simulink model "cx06_MA"  (Simulink 7.5)
settings: Solver=FixedStepDiscrete  StartTime=0.0  StopTime=10.0  RelTol=1e-3
undefined symbols (not defined in the file or in its folder): DiscIntNeverNeededParam, ECU555, int, motohawk_build_version, motohawk_trunc_name, motohawk_vardec_path
libraries: MotoHawk_lib x811, simulink x43, simulink_need_slupdate x1
(part 9 of 10)

== system cx06_MA/Inputs/Analog Inputs/Driver Inputs/Brake ==
  2pt Calibration1_1 : Fcn  Expr=(u[1]-u[2])/(u[3]-u[2])
  2pt Calibration1_6 : Fcn  Expr=(u[1]-u[2])/(u[3]-u[2])
  Data Type Conversion2 : DataTypeConversion  OutDataTypeMode=single  OutDataType=sfix(16)  OutScaling=2^0  OutDataTypeStr=single
  Data Type Conversion5 : DataTypeConversion  OutDataTypeMode=single  OutDataType=sfix(16)  OutScaling=2^0  OutDataTypeStr=single
  Mux3 : Mux  Inputs=3
  Mux6 : Mux  Inputs=3
  Range_Detect2 : Subsystem
  Range_Detect5 : Subsystem
  Redundant_Check : Subsystem
  Saturation2 : Saturate  UpperLimit=1  LowerLimit=0
  Saturation5 : Saturate  UpperLimit=1  LowerLimit=0
  motohawk_ain2 : MotoHawk_lib/Analog I//O Blocks/motohawk_ain  res_name=[]  text_resource=AN10M  code_resource=NONE  val_resource=-1  target=ECU555-80  resource_enum_str=(None)=-1,ECUP=53,DRVP=54,XDRP=55,AN1M=56,AN2M=57,AN3M=58,AN4M=59,AN5M=60,AN6M=61,AN7M=62,AN8M=63,AN9M=64,AN10M=65,AN11M=66,AN12M=67,AN13M=68,AN14M=69,AN15M=70,AN16M=71,AN17M=72,AN18M=73,AN19M=74,O2A=90,O2B=91,XDRP_B=92  altref=5V Reference  typ=uint16  num_adc_bits=10  use_stat=on  use_vardec=on  nam='Brake'  read_level=1  write_level=1  group='I/O Pins | Inputs Config'
  motohawk_ain6 : MotoHawk_lib/Analog I//O Blocks/motohawk_ain  res_name=[]  text_resource=AN7M  code_resource=NONE  val_resource=-1  target=ECU555-80  resource_enum_str=(None)=-1,ECUP=53,DRVP=54,XDRP=55,AN1M=56,AN2M=57,AN3M=58,AN4M=59,AN5M=60,AN6M=61,AN7M=62,AN8M=63,AN9M=64,AN10M=65,AN11M=66,AN12M=67,AN13M=68,AN14M=69,AN15M=70,AN16M=71,AN17M=72,AN18M=73,AN19M=74,O2A=90,O2B=91,XDRP_B=92  altref=5V Reference  typ=uint16  num_adc_bits=10  use_stat=on  use_vardec=on  nam='BrakeBackUp'  read_level=1  write_level=1  group='I/O Pins | Inputs Config'
  motohawk_calibration1 : MotoHawk_lib/Calibration & Probing Blocks/motohawk_calibration  nam='Brake_Redun_Err'  val=1  storage=Calibration  show_more=on  name_source=Use Parameter  data_type=Inherit via back propagation  read_level=1  write_level=1  ovr_cals=on  view_as=Number  enum_struct={'Disabled', 'Enabled'}  vector_style=Wide Row  use_help_units=on  help='Brake sensors must be within this error else Redundante Fault'  units=''  use_header_enum=off  row_header_enum={}  col_header_enum={}  use_min_max=on  min_val=0  max_val=1.2  use_precision=on  precision='1.2'  gain=1  offset=0  exp=1  use_mototune_group=off  mototune_group=motohawk_vardec_path(gcb)
  motohawk_calibration11 : MotoHawk_lib/Calibration & Probing Blocks/motohawk_calibration  nam='BrakeBackup_Full'  val=597  storage=Calibration  show_more=on  name_source=Use Parameter  data_type=Inherit via back propagation  read_level=1  write_level=1  ovr_cals=on  view_as=Number  enum_struct={'Disabled', 'Enabled'}  vector_style=Wide Row  use_help_units=off  help=''  units=''  use_header_enum=off  row_header_enum={}  col_header_enum={}  use_min_max=off  min_val=-inf  max_val=inf  use_precision=off  precision=''  gain=1  offset=0  exp=1  use_mototune_group=off  mototune_group=motohawk_vardec_path(gcb)
  motohawk_calibration12 : MotoHawk_lib/Calibration & Probing Blocks/motohawk_calibration  nam='BrakeBackup_Zero'  val=678  storage=Calibration  show_more=on  name_source=Use Parameter  data_type=Inherit via back propagation  read_level=1  write_level=1  ovr_cals=on  view_as=Number  enum_struct={'Disabled', 'Enabled'}  vector_style=Wide Row  use_help_units=off  help=''  units=''  use_header_enum=off  row_header_enum={}  col_header_enum={}  use_min_max=off  min_val=-inf  max_val=inf  use_precision=off  precision=''  gain=1  offset=0  exp=1  use_mototune_group=off  mototune_group=motohawk_vardec_path(gcb)
  motohawk_calibration5 : MotoHawk_lib/Calibration & Probing Blocks/motohawk_calibration  nam='Brake_Zero'  val=925  storage=Calibration  show_more=on  name_source=Use Parameter  data_type=Inherit via back propagation  read_level=1  write_level=1  ovr_cals=on  view_as=Number  enum_struct={'Disabled', 'Enabled'}  vector_style=Wide Row  use_help_units=off  help=''  units=''  use_header_enum=off  row_header_enum={}  col_header_enum={}  use_min_max=off  min_val=-inf  max_val=inf  use_precision=off  precision=''  gain=1  offset=0  exp=1  use_mototune_group=off  mototune_group=motohawk_vardec_path(gcb)
  motohawk_calibration6 : MotoHawk_lib/Calibration & Probing Blocks/motohawk_calibration  nam='Brake_Full'  val=37  storage=Calibration  show_more=on  name_source=Use Parameter  data_type=Inherit via back propagation  read_level=1  write_level=1  ovr_cals=on  view_as=Number  enum_struct={'Disabled', 'Enabled'}  vector_style=Wide Row  use_help_units=off  help=''  units=''  use_header_enum=off  row_header_enum={}  col_header_enum={}  use_min_max=off  min_val=-inf  max_val=inf  use_precision=off  precision=''  gain=1  offset=0  exp=1  use_mototune_group=off  mototune_group=motohawk_vardec_path(gcb)
  motohawk_fault_def1 : MotoHawk_lib/Fault Management Blocks/motohawk_fault_def  nam='BrakeRedundant'  mode=Disabled  id=[]  x=10  y=20  input_suspected=on  indeterminate=off  increment_xy=on  downsample_count=1  ovr_cals=on  ovr_actions=on  show_actions=on  action1_name='inhibitRegen'  action1_cond=Active  action2_name=''  action2_cond=(None)  action3_name=''  action3_cond=(None)  action4_name=''  action4_cond=(None)
  motohawk_fault_def3 : MotoHawk_lib/Fault Management Blocks/motohawk_fault_def  nam='BrakeRange'  mode=Disabled  id=[]  x=10  y=20  input_suspected=on  indeterminate=off  increment_xy=on  downsample_count=1  ovr_cals=on  ovr_actions=on  show_actions=on  action1_name='inhibitRegen'  action1_cond=Active  action2_name=''  action2_cond=(None)  action3_name=''  action3_cond=(None)  action4_name=''  action4_cond=(None)
  motohawk_fault_def6 : MotoHawk_lib/Fault Management Blocks/motohawk_fault_def  nam='BrakeBackupRange'  mode=Disabled  id=[]  x=10  y=20  input_suspected=on  indeterminate=off  increment_xy=on  downsample_count=1  ovr_cals=on  ovr_actions=on  show_actions=on  action1_name='inhibitRegen'  action1_cond=Active  action2_name=''  action2_cond=(None)  action3_name=''  action3_cond=(None)  action4_name=''  action4_cond=(None)
  motohawk_probe11 : MotoHawk_lib/Calibration & Probing Blocks/motohawk_probe  nam='In_Brake'  show_more=on  name_source=Use Parameter  read_level=1  view_as=Number  enum_struct={'Disabled', 'Enabled'}  vector_style=Wide Row  use_help_units=off  help=''  units=''  use_header_enum=off  row_header_enum={}  col_header_enum={}  use_precision=off  precision=''  gain=1  offset=0  exp=1  use_mototune_group=on  mototune_group='Debug | Inputs'
  motohawk_probe17 : MotoHawk_lib/Calibration & Probing Blocks/motohawk_probe  nam='In_BrakeBackup'  show_more=on  name_source=Use Parameter  read_level=1  view_as=Number  enum_struct={'Disabled', 'Enabled'}  vector_style=Wide Row  use_help_units=off  help=''  units=''  use_header_enum=off  row_header_enum={}  col_header_enum={}  use_precision=off  precision=''  gain=1  offset=0  exp=1  use_mototune_group=on  mototune_group='Debug | Inputs'
  motohawk_probe18 : MotoHawk_lib/Calibration & Probing Blocks/motohawk_probe  nam='raw_BrakeBackup'  show_more=on  name_source=Use Parameter  read_level=1  view_as=Number  enum_struct={'Disabled', 'Enabled'}  vector_style=Wide Row  use_help_units=on  help=''  units=''  use_header_enum=off  row_header_enum={}  col_header_enum={}  use_precision=off  precision=''  gain=1  offset=0  exp=1  use_mototune_group=off  mototune_group=motohawk_vardec_path(gcb)
  motohawk_probe19 : MotoHawk_lib/Calibration & Probing Blocks/motohawk_probe  nam='cal_BrakeBackup'  show_more=on  name_source=Use Parameter  read_level=1  view_as=Number  enum_struct={'Disabled', 'Enabled'}  vector_style=Wide Row  use_help_units=off  help=''  units=''  use_header_enum=off  row_header_enum={}  col_header_enum={}  use_precision=off  precision=''  gain=1  offset=0  exp=1  use_mototune_group=off  mototune_group=motohawk_vardec_path(gcb)
  motohawk_probe5 : MotoHawk_lib/Calibration & Probing Blocks/motohawk_probe  nam='raw_Brake'  show_more=on  name_source=Use Parameter  read_level=1  view_as=Number  enum_struct={'Disabled', 'Enabled'}  vector_style=Wide Row  use_help_units=on  help=''  units=''  use_header_enum=off  row_header_enum={}  col_header_enum={}  use_precision=off  precision=''  gain=1  offset=0  exp=1  use_mototune_group=off  mototune_group=motohawk_vardec_path(gcb)
  motohawk_probe6 : MotoHawk_lib/Calibration & Probing Blocks/motohawk_probe  nam='cal_Brake'  show_more=on  name_source=Use Parameter  read_level=1  view_as=Number  enum_struct={'Disabled', 'Enabled'}  vector_style=Wide Row  use_help_units=off  help=''  units=''  use_header_enum=off  row_header_enum={}  col_header_enum={}  use_precision=off  precision=''  gain=1  offset=0  exp=1  use_mototune_group=off  mototune_group=motohawk_vardec_path(gcb)
  Brake : Outport  OutDataType=sfix(16)  OutScaling=2^0
  wires:
  motohawk_ain2/1 -> motohawk_probe5/1, Data Type Conversion2/1
  motohawk_calibration5/1 -> Mux3/2, Range_Detect2/2(Zero)
  motohawk_calibration6/1 -> Mux3/3, Range_Detect2/3(Full)
  Mux3/1 -> 2pt Calibration1_1/1
  2pt Calibration1_1/1 -> Saturation2/1
  Data Type Conversion2/1 -> Mux3/1, Range_Detect2/1(Value)
  Saturation2/1 -> motohawk_probe6/1, Redundant_Check/1(In1), Brake/1  "Brake"
  Range_Detect2/1(Fault) -> motohawk_fault_def3/1
  motohawk_ain2/2 -> motohawk_probe11/1
  motohawk_ain6/1 -> Data Type Conversion5/1, motohawk_probe18/1
  motohawk_calibration12/1 -> Mux6/2, Range_Detect5/2(Zero)
  motohawk_calibration11/1 -> Mux6/3, Range_Detect5/3(Full)
  Mux6/1 -> 2pt Calibration1_6/1
  2pt Calibration1_6/1 -> Saturation5/1
  Data Type Conversion5/1 -> Mux6/1, Range_Detect5/1(Value)
  Saturation5/1 -> motohawk_probe19/1, Redundant_Check/3(In2)  "BrakeBackup"
  Range_Detect5/1(Fault) -> motohawk_fault_def6/1
  motohawk_ain6/2 -> motohawk_probe17/1
  motohawk_calibration1/1 -> Redundant_Check/2(Allowable_Error)
  Redundant_Check/1(Fault) -> motohawk_fault_def1/1

== system cx06_MA/Inputs/Analog Inputs/Driver Inputs/Clutch ==
  2pt Calibration1_4 : Fcn  Expr=(u[1]-u[2])/(u[3]-u[2])
  2pt Calibration1_5 : Fcn  Expr=(u[1]-u[2])/(u[3]-u[2])
  Data Type Conversion3 : DataTypeConversion  OutDataTypeMode=single  OutDataType=sfix(16)  OutScaling=2^0  OutDataTypeStr=single
  Data Type Conversion4 : DataTypeConversion  OutDataTypeMode=single  OutDataType=sfix(16)  OutScaling=2^0  OutDataTypeStr=single
  Mux4 : Mux  Inputs=3
  Mux5 : Mux  Inputs=3
  Range_Detect3 : Subsystem
  Range_Detect4 : Subsystem
  Redundant_Check : Subsystem
  Saturation3 : Saturate  UpperLimit=1  LowerLimit=0
  Saturation4 : Saturate  UpperLimit=1  LowerLimit=0
  motohawk_ain3 : MotoHawk_lib/Analog I//O Blocks/motohawk_ain  res_name=[]  text_resource=AN8M  code_resource=NONE  val_resource=-1  target=ECU555-80  resource_enum_str=(None)=-1,ECUP=53,DRVP=54,XDRP=55,AN1M=56,AN2M=57,AN3M=58,AN4M=59,AN5M=60,AN6M=61,AN7M=62,AN8M=63,AN9M=64,AN10M=65,AN11M=66,AN12M=67,AN13M=68,AN14M=69,AN15M=70,AN16M=71,AN17M=72,AN18M=73,AN19M=74,O2A=90,O2B=91,XDRP_B=92  altref=5V Reference  typ=uint16  num_adc_bits=10  use_stat=on  use_vardec=on  nam='Clutch'  read_level=1  write_level=1  group='I/O Pins | Inputs Config'
  motohawk_ain5 : MotoHawk_lib/Analog I//O Blocks/motohawk_ain  res_name=[]  text_resource=(None)  code_resource=NONE  val_resource=-1  target=ECU555-80  resource_enum_str=(None)=-1,ECUP=53,DRVP=54,XDRP=55,AN1M=56,AN2M=57,AN3M=58,AN4M=59,AN5M=60,AN6M=61,AN7M=62,AN8M=63,AN9M=64,AN10M=65,AN11M=66,AN12M=67,AN13M=68,AN14M=69,AN15M=70,AN16M=71,AN17M=72,AN18M=73,AN19M=74,O2A=90,O2B=91,XDRP_B=92  altref=5V Reference  typ=uint16  num_adc_bits=10  use_stat=on  use_vardec=on  nam='ClutchBackup'  read_level=1  write_level=1  group='I/O Pins | Inputs Config'
  motohawk_calibration1 : MotoHawk_lib/Calibration & Probing Blocks/motohawk_calibration  nam='Clutch_Redun_Err'  val=1  storage=Calibration  show_more=on  name_source=Use Parameter  data_type=Inherit via back propagation  read_level=1  write_level=1  ovr_cals=on  view_as=Number  enum_struct={'Disabled', 'Enabled'}  vector_style=Wide Row  use_help_units=on  help='Brake sensors must be within this error else Redundante Fault'  units=''  use_header_enum=off  row_header_enum={}  col_header_enum={}  use_min_max=on  min_val=0  max_val=1  use_precision=on  precision='1.2'  gain=1  offset=0  exp=1  use_mototune_group=off  mototune_group=motohawk_vardec_path(gcb)
  motohawk_calibration10 : MotoHawk_lib/Calibration & Probing Blocks/motohawk_calibration  nam='ClutchBackup_Full'  val=.75  storage=Calibration  show_more=on  name_source=Use Parameter  data_type=Inherit via back propagation  read_level=1  write_level=1  ovr_cals=on  view_as=Number  enum_struct={'Disabled', 'Enabled'}  vector_style=Wide Row  use_help_units=off  help=''  units=''  use_header_enum=off  row_header_enum={}  col_header_enum={}  use_min_max=off  min_val=-inf  max_val=inf  use_precision=off  precision=''  gain=1  offset=0  exp=1  use_mototune_group=off  mototune_group=motohawk_vardec_path(gcb)
  motohawk_calibration7 : MotoHawk_lib/Calibration & Probing Blocks/motohawk_calibration  nam='Clutch_Zero'  val=110  storage=Calibration  show_more=on  name_source=Use Parameter  data_type=Inherit via back propagation  read_level=1  write_level=1  ovr_cals=on  view_as=Number  enum_struct={'Disabled', 'Enabled'}  vector_style=Wide Row  use_help_units=off  help=''  units=''  use_header_enum=off  row_header_enum={}  col_header_enum={}  use_min_max=off  min_val=-inf  max_val=inf  use_precision=off  precision=''  gain=1  offset=0  exp=1  use_mototune_group=off  mototune_group=motohawk_vardec_path(gcb)
  motohawk_calibration8 : MotoHawk_lib/Calibration & Probing Blocks/motohawk_calibration  nam='Clutch_Full'  val=1015  storage=Calibration  show_more=on  name_source=Use Parameter  data_type=Inherit via back propagation  read_level=1  write_level=1  ovr_cals=on  view_as=Number  enum_struct={'Disabled', 'Enabled'}  vector_style=Wide Row  use_help_units=off  help=''  units=''  use_header_enum=off  row_header_enum={}  col_header_enum={}  use_min_max=off  min_val=-inf  max_val=inf  use_precision=off  precision=''  gain=1  offset=0  exp=1  use_mototune_group=off  mototune_group=motohawk_vardec_path(gcb)
  motohawk_calibration9 : MotoHawk_lib/Calibration & Probing Blocks/motohawk_calibration  nam='ClutchBackup_Zero'  val=.5  storage=Calibration  show_more=on  name_source=Use Parameter  data_type=Inherit via back propagation  read_level=1  write_level=1  ovr_cals=on  view_as=Number  enum_struct={'Disabled', 'Enabled'}  vector_style=Wide Row  use_help_units=off  help=''  units=''  use_header_enum=off  row_header_enum={}  col_header_enum={}  use_min_max=off  min_val=-inf  max_val=inf  use_precision=off  precision=''  gain=1  offset=0  exp=1  use_mototune_group=off  mototune_group=motohawk_vardec_path(gcb)
  motohawk_fault_def1 : MotoHawk_lib/Fault Management Blocks/motohawk_fault_def  nam='ClutchRedundant'  mode=Sticky  id=[]  x=10  y=20  input_suspected=on  indeterminate=off  increment_xy=on  downsample_count=1  ovr_cals=on  ovr_actions=on  show_actions=on  action1_name='inhibitEngineSS'  action1_cond=Active  action2_name='inhibitAssistTakeoff'  action2_cond=(None)  action3_name='Clutch'  action3_cond=(None)  action4_name=''  action4_cond=(None)
  motohawk_fault_def4 : MotoHawk_lib/Fault Management Blocks/motohawk_fault_def  nam='ClutchRange'  mode=Disabled  id=[]  x=10  y=20  input_suspected=on  indeterminate=off  increment_xy=on  downsample_count=1  ovr_cals=on  ovr_actions=on  show_actions=on  action1_name='inhibitEngineSS'  action1_cond=Active  action2_name='inhibitAssistTakeoff'  action2_cond=Active  action3_name='Clutch'  action3_cond=Active  action4_name=''  action4_cond=(None)
  motohawk_fault_def5 : MotoHawk_lib/Fault Management Blocks/motohawk_fault_def  nam='ClutchBackupRange'  mode=Disabled  id=[]  x=10  y=20  input_suspected=on  indeterminate=off  increment_xy=on  downsample_count=1  ovr_cals=on  ovr_actions=on  show_actions=on  action1_name='inhibitEngineSS'  action1_cond=Active  action2_name='inhibitAssistTakeoff'  action2_cond=Active  action3_name='Clutch'  action3_cond=Active  action4_name=''  action4_cond=(None)
  motohawk_probe12 : MotoHawk_lib/Calibration & Probing Blocks/motohawk_probe  nam='In_Clutch'  show_more=on  name_source=Use Parameter  read_level=1  view_as=Number  enum_struct={'Disabled', 'Enabled'}  vector_style=Wide Row  use_help_units=off  help=''  units=''  use_header_enum=off  row_header_enum={}  col_header_enum={}  use_precision=off  precision=''  gain=1  offset=0  exp=1  use_mototune_group=on  mototune_group='Debug | Inputs'
  motohawk_probe13 : MotoHawk_lib/Calibration & Probing Blocks/motohawk_probe  nam='In_ClutchBackup'  show_more=on  name_source=Use Parameter  read_level=1  view_as=Number  enum_struct={'Disabled', 'Enabled'}  vector_style=Wide Row  use_help_units=off  help=''  units=''  use_header_enum=off  row_header_enum={}  col_header_enum={}  use_precision=off  precision=''  gain=1  offset=0  exp=1  use_mototune_group=on  mototune_group='Debug | Inputs'
  motohawk_probe14 : MotoHawk_lib/Calibration & Probing Blocks/motohawk_probe  nam='raw_ClutchBackup'  show_more=on  name_source=Use Parameter  read_level=1  view_as=Number  enum_struct={'Disabled', 'Enabled'}  vector_style=Wide Row  use_help_units=on  help=''  units=''  use_header_enum=off  row_header_enum={}  col_header_enum={}  use_precision=off  precision=''  gain=1  offset=0  exp=1  use_mototune_group=off  mototune_group=motohawk_vardec_path(gcb)
  motohawk_probe15 : MotoHawk_lib/Calibration & Probing Blocks/motohawk_probe  nam='cal_ClutchBackup'  show_more=on  name_source=Use Parameter  read_level=1  view_as=Number  enum_struct={'Disabled', 'Enabled'}  vector_style=Wide Row  use_help_units=off  help=''  units=''  use_header_enum=off  row_header_enum={}  col_header_enum={}  use_precision=off  precision=''  gain=1  offset=0  exp=1  use_mototune_group=off  mototune_group=motohawk_vardec_path(gcb)
  motohawk_probe7 : MotoHawk_lib/Calibration & Probing Blocks/motohawk_probe  nam='raw_Clutch'  show_more=on  name_source=Use Parameter  read_level=1  view_as=Number  enum_struct={'Disabled', 'Enabled'}  vector_style=Wide Row  use_help_units=on  help=''  units=''  use_header_enum=off  row_header_enum={}  col_header_enum={}  use_precision=off  precision=''  gain=1  offset=0  exp=1  use_mototune_group=off  mototune_group=motohawk_vardec_path(gcb)
  motohawk_probe8 : MotoHawk_lib/Calibration & Probing Blocks/motohawk_probe  nam='cal_Clutch'  show_more=on  name_source=Use Parameter  read_level=1  view_as=Number  enum_struct={'Disabled', 'Enabled'}  vector_style=Wide Row  use_help_units=off  help=''  units=''  use_header_enum=off  row_header_enum={}  col_header_enum={}  use_precision=off  precision=''  gain=1  offset=0  exp=1  use_mototune_group=off  mototune_group=motohawk_vardec_path(gcb)
  Clutch : Outport  OutDataType=sfix(16)  OutScaling=2^0
  wires:
  motohawk_ain3/1 -> Data Type Conversion3/1, motohawk_probe7/1
  motohawk_calibration7/1 -> Mux4/2, Range_Detect3/2(Zero)
  motohawk_calibration8/1 -> Mux4/3, Range_Detect3/3(Full)
  Mux4/1 -> 2pt Calibration1_4/1
  2pt Calibration1_4/1 -> Saturation3/1
  Data Type Conversion3/1 -> Mux4/1, Range_Detect3/1(Value)
  Saturation3/1 -> motohawk_probe8/1, Redundant_Check/1(In1), Clutch/1  "Clutch"
  Range_Detect3/1(Fault) -> motohawk_fault_def4/1
  motohawk_ain3/2 -> motohawk_probe12/1
  motohawk_ain5/1 -> Data Type Conversion4/1, motohawk_probe14/1
  motohawk_calibration9/1 -> Mux5/2, Range_Detect4/2(Zero)
  motohawk_calibration10/1 -> Mux5/3, Range_Detect4/3(Full)
  Mux5/1 -> 2pt Calibration1_5/1
  2pt Calibration1_5/1 -> Saturation4/1
  Data Type Conversion4/1 -> Mux5/1, Range_Detect4/1(Value)
  Saturation4/1 -> motohawk_probe15/1, Redundant_Check/3(In2)  "ClutchBackup"
  Range_Detect4/1(Fault) -> motohawk_fault_def5/1
  motohawk_ain5/2 -> motohawk_probe13/1
  motohawk_calibration1/1 -> Redundant_Check/2(Allowable_Error)
  Redundant_Check/1(Fault) -> motohawk_fault_def1/1

== system cx06_MA/Inputs/Analog Inputs/Fuel Level/Range_Detect ==
  Value : Inport  OutDataType=sfix(16)  OutScaling=2^0
  Zero : Inport  Port=2  OutDataType=sfix(16)  OutScaling=2^0
  Full : Inport  Port=3  OutDataType=sfix(16)  OutScaling=2^0
  Gain : Gain  Gain=0.1  ParameterDataType=sfix(16)  ParameterScaling=2^0  OutDataType=sfix(16)  OutScaling=2^0
  Logical Operator : Logic  Operator=OR  AllPortsSameDT=off  OutDataTypeMode=boolean  OutDataTypeStr=boolean
  MinMax : MinMax  Inputs=2  OutDataType=sfix(16)  OutScaling=2^0
  MinMax1 : MinMax  Function=max  Inputs=2  OutDataType=sfix(16)  OutScaling=2^0
  Relational Operator : RelationalOperator  Operator=>  LogicOutDataTypeMode=boolean  OutDataTypeStr=boolean
  Relational Operator1 : RelationalOperator  Operator=>  LogicOutDataTypeMode=boolean  OutDataTypeStr=boolean
  Sum : Sum  Inputs=|+-  OutDataType=sfix(16)  OutScaling=2^0
  Sum1 : Sum  Inputs=-+  OutDataType=sfix(16)  OutScaling=2^0
  Sum2 : Sum  Inputs=++|  OutDataType=sfix(16)  OutScaling=2^0
  Fault : Outport  OutDataType=sfix(16)  OutScaling=2^0
  wires:
  Zero/1 -> MinMax/1, MinMax1/2
  Full/1 -> MinMax/2, MinMax1/1
  MinMax/1 -> Sum1/1, Sum/1
  MinMax1/1 -> Sum1/2, Sum2/2
  Sum1/1 -> Gain/1
  Gain/1 -> Sum/2, Sum2/1
  Sum2/1 -> Relational Operator1/2
  Sum/1 -> Relational Operator/1
  Value/1 -> Relational Operator/2, Relational Operator1/1
  Relational Operator/1 -> Logical Operator/1
  Relational Operator1/1 -> Logical Operator/2
  Logical Operator/1 -> Fault/1

== system cx06_MA/Outputs/Analog Outputs/Backup_Relay_Control/Subsystem ==
  timer_en : Inport  OutDataType=sfix(16)  OutScaling=2^0
  Idle_to_Crank Cal : Inport  Port=2  OutDataType=sfix(16)  OutScaling=2^0
  Crank_to_Idle Cal : Inport  Port=3  OutDataType=sfix(16)  OutScaling=2^0
  Constant : Constant  Value=0  OutDataType=sfix(16)  OutScaling=2^0
  Constant1 : Constant  OutDataType=sfix(16)  OutScaling=2^0
  Relational Operator : RelationalOperator  LogicOutDataTypeMode=boolean  OutDataTypeStr=boolean
  Relational Operator1 : RelationalOperator  Operator=<=  LogicOutDataTypeMode=boolean  OutDataTypeStr=boolean
  Saturation : Saturate  UpperLimit=300  LowerLimit=0
  Sum : Sum  Inputs=|++  OutDataType=sfix(16)  OutScaling=2^0
  Switch1 : Switch  Criteria=u2 > Threshold  OutDataTypeStr=Inherit: Inherit via back propagation
  Unit Delay : UnitDelay  SampleTime=-1
  Timer : Outport  OutDataType=sfix(16)  OutScaling=2^0
  Idle_to_Crank Delay : Outport  Port=2  OutDataType=sfix(16)  OutScaling=2^0
  Crank_to_Idle Delay : Outport  Port=3  OutDataType=sfix(16)  OutScaling=2^0
  wires:
  Switch1/1 -> Saturation/1
  Saturation/1 -> Timer/1, Relational Operator/1, Unit Delay/1, Relational Operator1/2
  Constant/1 -> Switch1/3
  Constant1/1 -> Sum/2
  Sum/1 -> Switch1/1
  timer_en/1 -> Switch1/2
  Crank_to_Idle Cal/1 -> Relational Operator/2
  Relational Operator/1 -> Crank_to_Idle Delay/1
  Idle_to_Crank Cal/1 -> Relational Operator1/1
  Relational Operator1/1 -> Idle_to_Crank Delay/1
  Unit Delay/1 -> Sum/1

== system cx06_MA/Outputs/GMLAN Outputs/Fuel/SOC_Gage_Conditioning/Fuel_Signal_Conditioning ==
  note: Regular Filter to keep fuel gage from "bouncing" around;
      | also, on start up, it passes though the unfiltered value
  Fuel_Level : Inport  OutDataType=sfix(16)  OutScaling=2^0
  Constant : Constant  OutDataType=sfix(16)  OutScaling=2^0
  Gain : Gain  Gain=100  ParameterDataType=sfix(16)  ParameterScaling=2^0  OutDataType=sfix(16)  OutScaling=2^0
  Product : Product  OutDataType=sfix(16)  OutScaling=2^0  RndMeth=Zero
  Product1 : Product  OutDataType=sfix(16)  OutScaling=2^0  RndMeth=Zero
  Sum : Sum  Inputs=|++  OutDataType=sfix(16)  OutScaling=2^0
  Sum1 : Sum  Inputs=|-+  OutDataType=sfix(16)  OutScaling=2^0
  Switch : Switch  Criteria=u2 > Threshold  Threshold=-1
  Unit Delay1 : UnitDelay  X0=-1  SampleTime=-1
  motohawk_calibration : MotoHawk_lib/Calibration & Probing Blocks/motohawk_calibration  nam='Fuel_Filter_K'  val=.0001  storage=Calibration  show_more=on  name_source=Use Parameter  data_type=Inherit from 'Default Value'  read_level=1  write_level=1  ovr_cals=on  view_as=Number  enum_struct={'Disabled', 'Enabled'}  vector_style=Wide Row  use_help_units=off  help=''  units=''  use_header_enum=off  row_header_enum={}  col_header_enum={}  use_min_max=on  min_val=0  max_val=1  use_precision=on  precision='1.4'  gain=1  offset=0  exp=1  use_mototune_group=off  mototune_group=motohawk_vardec_path(gcb)
  Out1 : Outport  OutDataType=sfix(16)  OutScaling=2^0
  wires:
  motohawk_calibration/1 -> Product/2, Sum1/1
  Product/1 -> Sum/1
  Constant/1 -> Sum1/2
  Sum1/1 -> Product1/1
  Product1/1 -> Sum/2
  Unit Delay1/1 -> Product1/2, Switch/2
  Sum/1 -> Switch/1
  Gain/1 -> Product/1, Switch/3
  Switch/1 -> Out1/1, Unit Delay1/1
  Fuel_Level/1 -> Gain/1

== system cx06_MA/Strategy/Hybrid Control Code/Activation of Traction Control/RRef_Wheel Diff ==
  Inputs : Inport  OutDataType=sfix(16)  OutScaling=2^0
  Action Port : ActionPort  ActionType=case
  Abs{1..4} (4 alike) : Abs
  Bus Selector : BusSelector  OutputSignals=GMLAN.FL_Whl_Spd,GMLAN.FR_Whl_Spd,GMLAN.RL_Whl_Spd,GMLAN.RR_Whl_Spd
  Logical Operator : Logic  Operator=OR  AllPortsSameDT=off  OutDataTypeMode=Specify via dialog  OutDataTypeStr=uint(8)
  MinMax : MinMax  Inputs=2  OutDataType=sfix(16)  OutScaling=2^0
  MinMax1 : MinMax  Function=max  Inputs=2  OutDataType=sfix(16)  OutScaling=2^0
  MinMax2 : MinMax  Function=max  Inputs=2  OutDataType=sfix(16)  OutScaling=2^0
  MinMax3 : MinMax  Inputs=2  OutDataType=sfix(16)  OutScaling=2^0
  Relational Operator1 : RelationalOperator  Operator=>  LogicOutDataTypeMode=Specify via dialog  OutDataTypeStr=uint(8)
  Relational Operator2 : RelationalOperator  Operator=>  LogicOutDataTypeMode=Specify via dialog  OutDataTypeStr=uint(8)
  Relational Operator3 : RelationalOperator  Operator=>  LogicOutDataTypeMode=Specify via dialog  OutDataTypeStr=uint(8)
  Sum1 : Sum  Inputs=+-  OutDataType=sfix(16)  OutScaling=2^0
  Sum2 : Sum  Inputs=-+  OutDataType=sfix(16)  OutScaling=2^0
  Sum3 : Sum  Inputs=+-  OutDataType=sfix(16)  OutScaling=2^0
  motohawk_calibration : MotoHawk_lib/Calibration & Probing Blocks/motohawk_calibration  nam='TC_Slip_Thres'  val=10  storage=Calibration  show_more=on  name_source=Use Parameter  data_type=Inherit from 'Default Value'  read_level=1  write_level=1  ovr_cals=on  view_as=Number  enum_struct={'Disabled', 'Enabled'}  vector_style=Wide Row  use_help_units=on  help='max allowable wheel spd difference before TC become active'  units='rpm'  use_header_enum=off  row_header_enum={}  col_header_enum={}  use_min_max=on  min_val=0  max_val=inf  use_precision=off  precision=''  gain=1  offset=0  exp=1  use_mototune_group=off  mototune_group=motohawk_vardec_path(gcb)
  Front_Slip? : Outport  OutDataType=sfix(16)  OutScaling=2^0
  Rear_Slip? : Outport  Port=2  OutDataType=sfix(16)  OutScaling=2^0
  wires:
  Inputs/1 -> Bus Selector/1
  Bus Selector/3 -> Abs1/1  "<RL_Whl_Spd>"
  Bus Selector/4 -> Abs2/1  "<RR_Whl_Spd>"
  Abs1/1 -> MinMax/1
  Abs2/1 -> MinMax/2, MinMax2/1, MinMax2/2
  Bus Selector/2 -> Abs3/1  "<FR_Whl_Spd>"
  MinMax/1 -> Sum1/2, Sum2/1
  Bus Selector/1 -> Abs4/1  "<FL_Whl_Spd>"
  Sum1/1 -> Relational Operator2/1
  motohawk_calibration/1 -> Relational Operator2/2, Relational Operator1/2, Relational Operator3/2
  Relational Operator2/1 -> Front_Slip?/1
  Abs4/1 -> MinMax1/1, MinMax3/1
  Abs3/1 -> MinMax1/2, MinMax3/2
  MinMax1/1 -> Sum1/1
  MinMax2/1 -> Sum2/2, Sum3/1
  Sum2/1 -> Relational Operator1/1
  Logical Operator/1 -> Rear_Slip?/1
  MinMax3/1 -> Sum3/2
  Sum3/1 -> Relational Operator3/1
  Relational Operator3/1 -> Logical Operator/2
  Relational Operator1/1 -> Logical Operator/1

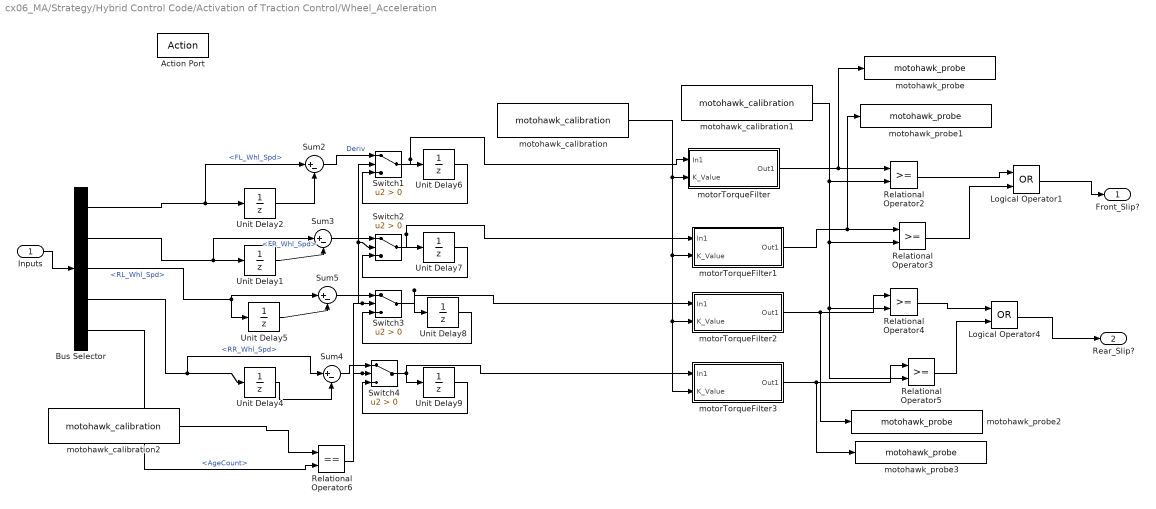
== system cx06_MA/Strategy/Hybrid Control Code/Activation of Traction Control/Wheel_Acceleration ==
  Inputs : Inport  OutDataType=sfix(16)  OutScaling=2^0
  Action Port : ActionPort  ActionType=case
  Bus Selector : BusSelector  OutputSignals=GMLAN.FL_Whl_Spd,GMLAN.FR_Whl_Spd,GMLAN.RL_Whl_Spd,GMLAN.RR_Whl_Spd,GMLAN.AgeCount
  Logical Operator1 : Logic  Operator=OR  AllPortsSameDT=off  OutDataTypeMode=Specify via dialog  OutDataTypeStr=uint(8)
  Logical Operator4 : Logic  Operator=OR  AllPortsSameDT=off  OutDataTypeMode=Specify via dialog  OutDataTypeStr=uint(8)
  Relational Operator{2..5} (4 alike) : RelationalOperator  LogicOutDataTypeMode=boolean  OutDataTypeStr=boolean
  Relational Operator6 : RelationalOperator  Operator===  LogicOutDataTypeMode=Specify via dialog  OutDataTypeStr=uint(8)
  Sum{2..5} (4 alike) : Sum  Inputs=|+-  OutDataType=sfix(16)  OutScaling=2^0
  Switch{1..4} (4 alike) : Switch  Criteria=u2 > Threshold
  Unit Delay{1..2,4..9} (8 alike) : UnitDelay  SampleTime=-1
  motohawk_calibration : MotoHawk_lib/Calibration & Probing Blocks/motohawk_calibration  nam='Filt_Wheel_Derv_K'  val=.02  storage=Calibration  show_more=on  name_source=Use Parameter  data_type=Inherit from 'Default Value'  read_level=1  write_level=1  ovr_cals=on  view_as=Number  enum_struct={'Disabled', 'Enabled'}  vector_style=Wide Row  use_help_units=off  help=''  units=''  use_header_enum=off  row_header_enum={}  col_header_enum={}  use_min_max=on  min_val=0  max_val=1  use_precision=on  precision='1.4'  gain=1  offset=0  exp=1  use_mototune_group=off  mototune_group=motohawk_vardec_path(gcb)
  motohawk_calibration1 : MotoHawk_lib/Calibration & Probing Blocks/motohawk_calibration  nam='TC_Accel_Thres'  val=6.5  storage=Calibration  show_more=on  name_source=Use Parameter  data_type=Inherit from 'Default Value'  read_level=1  write_level=1  ovr_cals=on  view_as=Number  enum_struct={'Disabled', 'Enabled'}  vector_style=Wide Row  use_help_units=on  help='wheel acceleration threshold for determining slip'  units='delta_rpm'  use_header_enum=off  row_header_enum={}  col_header_enum={}  use_min_max=on  min_val=0  max_val=inf  use_precision=off  precision=''  gain=1  offset=0  exp=1  use_mototune_group=off  mototune_group=motohawk_vardec_path(gcb)
  motohawk_calibration2 : MotoHawk_lib/Calibration & Probing Blocks/motohawk_calibration  nam='Age_Count_Comparison'  val=0  storage=Calibration  show_more=on  name_source=Use Parameter  data_type=Inherit from 'Default Value'  read_level=1  write_level=1  ovr_cals=on  view_as=Number  enum_struct={'Disabled', 'Enabled'}  vector_style=Wide Row  use_help_units=on  help='value that age_count must equal before wheel derivative is calculated'  units=''  use_header_enum=off  row_header_enum={}  col_header_enum={}  use_min_max=on  min_val=0  max_val=inf  use_precision=off  precision=''  gain=1  offset=0  exp=1  use_mototune_group=off  mototune_group=motohawk_vardec_path(gcb)
  motohawk_probe : MotoHawk_lib/Calibration & Probing Blocks/motohawk_probe  nam='Current_Derivative_Front_Left'  show_more=on  name_source=Use Parameter  read_level=1  view_as=Number  enum_struct={'Disabled', 'Enabled'}  vector_style=Wide Row  use_help_units=off  help=''  units=''  use_header_enum=off  row_header_enum={}  col_header_enum={}  use_precision=off  precision=''  gain=1  offset=0  exp=1  use_mototune_group=off  mototune_group=motohawk_vardec_path(gcb)
  motohawk_probe1 : MotoHawk_lib/Calibration & Probing Blocks/motohawk_probe  nam='Current_Derivative_Front_Right'  show_more=on  name_source=Use Parameter  read_level=1  view_as=Number  enum_struct={'Disabled', 'Enabled'}  vector_style=Wide Row  use_help_units=off  help=''  units=''  use_header_enum=off  row_header_enum={}  col_header_enum={}  use_precision=off  precision=''  gain=1  offset=0  exp=1  use_mototune_group=off  mototune_group=motohawk_vardec_path(gcb)
  motohawk_probe2 : MotoHawk_lib/Calibration & Probing Blocks/motohawk_probe  nam='Current_Derivative_Rear_Left'  show_more=on  name_source=Use Parameter  read_level=1  view_as=Number  enum_struct={'Disabled', 'Enabled'}  vector_style=Wide Row  use_help_units=off  help=''  units=''  use_header_enum=off  row_header_enum={}  col_header_enum={}  use_precision=off  precision=''  gain=1  offset=0  exp=1  use_mototune_group=off  mototune_group=motohawk_vardec_path(gcb)
  motohawk_probe3 : MotoHawk_lib/Calibration & Probing Blocks/motohawk_probe  nam='Current_Derivative_Rear_Right'  show_more=on  name_source=Use Parameter  read_level=1  view_as=Number  enum_struct={'Disabled', 'Enabled'}  vector_style=Wide Row  use_help_units=off  help=''  units=''  use_header_enum=off  row_header_enum={}  col_header_enum={}  use_precision=off  precision=''  gain=1  offset=0  exp=1  use_mototune_group=off  mototune_group=motohawk_vardec_path(gcb)
  motorTorqueFilter : Subsystem
  motorTorqueFilter1 : Subsystem
  motorTorqueFilter2 : Subsystem
  motorTorqueFilter3 : Subsystem
  Front_Slip? : Outport  OutDataType=sfix(16)  OutScaling=2^0
  Rear_Slip? : Outport  Port=2  OutDataType=sfix(16)  OutScaling=2^0
  wires:
  Inputs/1 -> Bus Selector/1
  Bus Selector/3 -> Unit Delay5/1, Sum5/1  "<RL_Whl_Spd>"
  motohawk_calibration1/1 -> Relational Operator2/2, Relational Operator3/2, Relational Operator4/2, Relational Operator5/2
  Unit Delay2/1 -> Sum2/2
  Unit Delay1/1 -> Sum3/2
  Unit Delay4/1 -> Sum4/2
  Unit Delay5/1 -> Sum5/2
  Relational Operator2/1 -> Logical Operator1/1
  Relational Operator3/1 -> Logical Operator1/2
  Relational Operator4/1 -> Logical Operator4/1
  Relational Operator5/1 -> Logical Operator4/2
  Bus Selector/1 -> Unit Delay2/1, Sum2/1  "<FL_Whl_Spd>"
  Bus Selector/2 -> Unit Delay1/1, Sum3/1  "<FR_Whl_Spd>"
  Bus Selector/4 -> Unit Delay4/1, Sum4/1  "<RR_Whl_Spd>"
  Bus Selector/5 -> Relational Operator6/2  "<AgeCount>"
  motohawk_calibration2/1 -> Relational Operator6/1
  Sum2/1 -> Switch1/1  "Deriv"
  Switch1/1 -> Unit Delay6/1, motorTorqueFilter/1(In1)
  Relational Operator6/1 -> Switch1/2, Switch2/2, Switch3/2, Switch4/2
  Unit Delay6/1 -> Switch1/3
  Logical Operator1/1 -> Front_Slip?/1
  Logical Operator4/1 -> Rear_Slip?/1
  Sum3/1 -> Switch2/1
  Switch2/1 -> Unit Delay7/1, motorTorqueFilter1/1(In1)
  Unit Delay7/1 -> Switch2/3
  Sum5/1 -> Switch3/1
  Switch3/1 -> Unit Delay8/1, motorTorqueFilter2/1(In1)
  Unit Delay8/1 -> Switch3/3
  Sum4/1 -> Switch4/1
  Switch4/1 -> Unit Delay9/1, motorTorqueFilter3/1(In1)
  Unit Delay9/1 -> Switch4/3
  motorTorqueFilter/1(Out1) -> Relational Operator2/1, motohawk_probe/1
  motorTorqueFilter1/1(Out1) -> Relational Operator3/1, motohawk_probe1/1
  motorTorqueFilter2/1(Out1) -> Relational Operator4/1, motohawk_probe2/1
  motorTorqueFilter3/1(Out1) -> Relational Operator5/1, motohawk_probe3/1
  motohawk_calibration/1 -> motorTorqueFilter/2(K_Value), motorTorqueFilter1/2(K_Value), motorTorqueFilter2/2(K_Value), motorTorqueFilter3/2(K_Value)

== system cx06_MA/Strategy/Hybrid Control Code/Engine Start-Stop/New_Alg ==
  In1 : Inport  OutDataType=sfix(16)  OutScaling=2^0
  Bus Creator : BusCreator  Inputs=9
  Bus Selector4 : BusSelector  OutputSignals=signal1,signal2,signal3,signal4,signal5,signal6,signal7,Neutral,running
  EngineSS_StateMachine1 : Stateflow chart  TreatAsAtomicUnit=on
  Out1 : Outport  OutDataType=sfix(16)  OutScaling=2^0
  wires:
  In1/1 -> Bus Selector4/1
  Bus Selector4/1 -> EngineSS_StateMachine1/1(clutching)  "<signal1>"
  Bus Selector4/2 -> EngineSS_StateMachine1/2(KillDelay)  "<signal2>"
  Bus Selector4/3 -> EngineSS_StateMachine1/3(Kill_Time)  "<signal3>"
  Bus Selector4/4 -> EngineSS_StateMachine1/4(Max_RetryCnt)  "<signal4>"
  Bus Selector4/5 -> EngineSS_StateMachine1/5(StartRetry_Delay)  "<signal5>"
  Bus Selector4/6 -> EngineSS_StateMachine1/6(Start_Delay)  "<signal6>"
  Bus Selector4/7 -> EngineSS_StateMachine1/7(Start_Time)  "<signal7>"
  Bus Selector4/8 -> EngineSS_StateMachine1/8(neutral)  "<Neutral>"
  Bus Selector4/9 -> EngineSS_StateMachine1/9(running)  "<running>"
  EngineSS_StateMachine1/1(KillDelay_Cnt) -> Bus Creator/1
  EngineSS_StateMachine1/2(Kill_Cnt) -> Bus Creator/2
  EngineSS_StateMachine1/3(StartDelay_Cnt) -> Bus Creator/3
  EngineSS_StateMachine1/5(StartRetry_Cnt) -> Bus Creator/5
  EngineSS_StateMachine1/6(Start_Cnt) -> Bus Creator/6
  Bus Creator/1 -> Out1/1
  EngineSS_StateMachine1/4(StartRetryDelay_Cnt) -> Bus Creator/4
  EngineSS_StateMachine1/7(kill) -> Bus Creator/7
  EngineSS_StateMachine1/8(start) -> Bus Creator/8
  EngineSS_StateMachine1/9(ESS_State) -> Bus Creator/9

== system cx06_MA/Strategy/Hybrid Control Code/Engine Start-Stop/Old_Alg ==
  In1 : Inport  OutDataType=sfix(16)  OutScaling=2^0
  Bus Creator : BusCreator  Inputs=9
  Bus Selector4 : BusSelector  OutputSignals=signal1,signal2,signal3,signal4,signal5,signal6,signal7,Neutral,running
  EngineSS_StateMachine : Stateflow chart  TreatAsAtomicUnit=on
  Out1 : Outport  OutDataType=sfix(16)  OutScaling=2^0
  wires:
  Bus Creator/1 -> Out1/1
  EngineSS_StateMachine/8(start) -> Bus Creator/8
  EngineSS_StateMachine/7(kill) -> Bus Creator/7
  EngineSS_StateMachine/6(Start_Cnt) -> Bus Creator/6
  EngineSS_StateMachine/5(StartRetry_Cnt) -> Bus Creator/5
  EngineSS_StateMachine/4(StartRetryDelay_Cnt) -> Bus Creator/4
  Bus Selector4/9 -> EngineSS_StateMachine/9(running)  "<running>"
  Bus Selector4/8 -> EngineSS_StateMachine/8(neutral)  "<Neutral>"
  Bus Selector4/7 -> EngineSS_StateMachine/7(Start_Time)  "<signal7>"
  Bus Selector4/6 -> EngineSS_StateMachine/6(Start_Delay)  "<signal6>"
  Bus Selector4/5 -> EngineSS_StateMachine/5(StartRetry_Delay)  "<signal5>"
  Bus Selector4/4 -> EngineSS_StateMachine/4(Max_RetryCnt)  "<signal4>"
  Bus Selector4/3 -> EngineSS_StateMachine/3(Kill_Time)  "<signal3>"
  Bus Selector4/2 -> EngineSS_StateMachine/2(KillDelay)  "<signal2>"
  Bus Selector4/1 -> EngineSS_StateMachine/1(clutching)  "<signal1>"
  In1/1 -> Bus Selector4/1
  EngineSS_StateMachine/9(ESS_State) -> Bus Creator/9
  EngineSS_StateMachine/1(KillDelay_Cnt) -> Bus Creator/1
  EngineSS_StateMachine/2(Kill_Cnt) -> Bus Creator/2
  EngineSS_StateMachine/3(StartDelay_Cnt) -> Bus Creator/3

== system cx06_MA/Strategy/Hybrid Control Code/HEV/AssistedTakeOff ==
  T_in : Inport  OutDataType=sfix(16)  OutScaling=2^0
  Inputs : Inport  Port=2  OutDataType=sfix(16)  OutScaling=2^0
  Activate? : Inport  Port=3  OutDataType=sfix(16)  OutScaling=2^0
  Bus Selector : BusSelector  OutputSignals=Analog.Driver.Clutch
  Bus Selector1 : BusSelector  OutputSignals=Analog.Driver.Clutch
  Bus Selector2 : BusSelector  OutputSignals=Analog.Driver.Clutch
  Constant : Constant  Value=0  OutDataType=sfix(16)  OutScaling=2^0
  Divide : Product  Inputs=/**  OutDataType=sfix(16)  OutScaling=2^-10
  Divide1 : Product  Inputs=*/*  OutDataType=sfix(16)  OutScaling=2^-10
  Divide2 : Product  Inputs=*/  OutDataType=sfix(16)  OutScaling=2^-10
  Embedded MATLAB Function : Stateflow chart  TreatAsAtomicUnit=on
  Logical Operator : Logic  Operator=NOT  AllPortsSameDT=off  OutDataTypeMode=boolean  OutDataTypeStr=boolean
  MinMax : MinMax  Function=max  Inputs=2  OutDataType=sfix(16)  OutScaling=2^0
  Multiport Switch : MultiPortSwitch  Inputs=5  zeroidx=off
  Product : Product  OutDataType=sfix(16)  OutScaling=2^0  RndMeth=Zero
  Product1 : Product  Inputs=3  OutDataType=sfix(16)  OutScaling=2^0  RndMeth=Zero
  Saturation : Saturate  UpperLimit=1  LowerLimit=0
  Sum : Sum  Inputs=+-  OutDataType=sfix(16)  OutScaling=2^0
  Sum1 : Sum  Inputs=-+  OutDataType=sfix(16)  OutScaling=2^0
  Sum2 : Sum  Inputs=+-  OutDataType=sfix(16)  OutScaling=2^0
  Sum3 : Sum  Inputs=-+  OutDataType=sfix(16)  OutScaling=2^0
  Sum4 : Sum  Inputs=|+-  OutDataType=sfix(16)  OutScaling=2^0
  Sum5 : Sum  Inputs=|-+  OutDataType=sfix(16)  OutScaling=2^0
  Sum6 : Sum  Inputs=|++  OutDataType=sfix(16)  OutScaling=2^0
  Switch : Switch  Criteria=u2 > Threshold
  motohawk_calibration : MotoHawk_lib/Calibration & Probing Blocks/motohawk_calibration  nam='AT_Full'  val=.75  storage=Calibration  show_more=on  name_source=Use Parameter  data_type=Inherit from 'Default Value'  read_level=1  write_level=1  ovr_cals=on  view_as=Number  enum_struct={'Disabled', 'Enabled'}  vector_style=Wide Row  use_help_units=on  help='Clutch Position where full assist is reached'  units='%'  use_header_enum=off  row_header_enum={}  col_header_enum={}  use_min_max=off  min_val=0  max_val=1  use_precision=on  precision='1.3'  gain=1  offset=0  exp=1  use_mototune_group=off  mototune_group=motohawk_vardec_path(gcb)
  motohawk_calibration1 : MotoHawk_lib/Calibration & Probing Blocks/motohawk_calibration  nam='AT_Ramp'  val=.55  storage=Calibration  show_more=on  name_source=Use Parameter  data_type=Inherit from 'Default Value'  read_level=1  write_level=1  ovr_cals=on  view_as=Number  enum_struct={'Disabled', 'Enabled'}  vector_style=Wide Row  use_help_units=on  help='Clutch Position where assist starts to ramp out'  units='%'  use_header_enum=off  row_header_enum={}  col_header_enum={}  use_min_max=off  min_val=0  max_val=1  use_precision=on  precision='1.3'  gain=1  offset=0  exp=1  use_mototune_group=off  mototune_group=motohawk_vardec_path(gcb)
  motohawk_calibration2 : MotoHawk_lib/Calibration & Probing Blocks/motohawk_calibration  nam='AT_Stop'  val=.5  storage=Calibration  show_more=on  name_source=Use Parameter  data_type=Inherit from 'Default Value'  read_level=1  write_level=1  ovr_cals=on  view_as=Number  enum_struct={'Disabled', 'Enabled'}  vector_style=Wide Row  use_help_units=on  help='Clutch Position where assist is gone'  units='%'  use_header_enum=off  row_header_enum={}  col_header_enum={}  use_min_max=off  min_val=0  max_val=1  use_precision=on  precision='1.3'  gain=1  offset=0  exp=1  use_mototune_group=off  mototune_group=motohawk_vardec_path(gcb)
  motohawk_calibration3 : MotoHawk_lib/Calibration & Probing Blocks/motohawk_calibration  nam='AT_Level'  val=.2  storage=Calibration  show_more=on  name_source=Use Parameter  data_type=Inherit from 'Default Value'  read_level=1  write_level=1  ovr_cals=on  view_as=Number  enum_struct={'Disabled', 'Enabled'}  vector_style=Wide Row  use_help_units=on  help='Max Assist Level'  units='%'  use_header_enum=off  row_header_enum={}  col_header_enum={}  use_min_max=off  min_val=0  max_val=1  use_precision=on  precision='1.3'  gain=1  offset=0  exp=1  use_mototune_group=off  mototune_group=motohawk_vardec_path(gcb)
  motohawk_data_def2 : MotoHawk_lib/Data Storage Blocks/motohawk_data_def  nam='AT_Start'  container_nam=''  data=0.75  typ=double  struct_nam='MyStruct'  storage=NonVolatile  outputRef=off  use_vardec=on  window=Calibration  read_level=1  write_level=1  ovr_cals=off  view_as=Number  enum_struct={'Disabled', 'Enabled'}  vector_style=Wide Row  use_help_units=on  help='AT Torque starts ramping in here'  units='%'  use_header_enum=off  row_header_enum=''  col_header_enum=''  use_min_max=off  min_val=0  max_val=1  use_precision=on  precision='1.2'  gain=1  offset=0  exp=1  use_mototune_group=off  mototune_group=motohawk_vardec_path(gcb)  eval_name=AT_Start  data_stores=motohawk_sfun_data_def_data_stores  struct_instances=motohawk_sfun_data_def_struct_instances  vardecs=motohawk_sfun_data_def_vardecs
  motohawk_data_read : MotoHawk_lib/Data Storage Blocks/motohawk_data_read  source=Lookup By Name  structure=Scalar  operation=Read scalar from location by index  sz_vec=4  sz_row=2  sz_col=3  typ=double  nam='AT_Start'  checkNull=on  struct_inst_name='Struct1'  struct_nam='MyStruct'
  motohawk_fault_action : MotoHawk_lib/Fault Management Blocks/motohawk_fault_action  nam='inhibitAssistTakeoff'  output_status=on  eval_nam=inhibitAssistTakeoff
  motohawk_probe1 : MotoHawk_lib/Calibration & Probing Blocks/motohawk_probe  nam='AT_TLevel'  show_more=on  name_source=Use Parameter  read_level=1  view_as=Number  enum_struct={'False', 'True'}  vector_style=Wide Row  use_help_units=off  help=''  units=''  use_header_enum=off  row_header_enum={}  col_header_enum={}  use_precision=on  precision='1.3'  gain=1  offset=0  exp=1  use_mototune_group=off  mototune_group=motohawk_vardec_path(gcb)
  T_Out : Outport  OutDataType=sfix(16)  OutScaling=2^0
  wires:
  motohawk_calibration/1 -> Sum/1, Embedded MATLAB Function/3(full)
  motohawk_data_read/1 -> Sum/2, Sum1/1, Embedded MATLAB Function/2(start)
  Inputs/1 -> Bus Selector/1, Bus Selector2/1, Bus Selector1/1
  Bus Selector/1 -> Sum1/2  "<Clutch>"
  Sum/1 -> Divide/1
  Sum1/1 -> Divide/2
  motohawk_calibration3/1 -> Divide1/1, Divide/3, Multiport Switch/4
  motohawk_calibration1/1 -> Sum2/1, Embedded MATLAB Function/4(ramp), Sum5/1, Sum4/2
  motohawk_calibration2/1 -> Sum2/2, Sum3/1, Embedded MATLAB Function/5(stop), Sum5/2
  Bus Selector1/1 -> Sum3/2  "<Clutch>"
  Sum2/1 -> Divide1/2
  Sum3/1 -> Divide1/3
  Divide/1 -> Multiport Switch/3
  Divide1/1 -> Multiport Switch/5
  Constant/1 -> Multiport Switch/6, Multiport Switch/2
  Embedded MATLAB Function/1(sw) -> Multiport Switch/1
  Bus Selector2/1 -> Embedded MATLAB Function/1(clutch), Sum4/1  "<Clutch>"
  Sum4/1 -> Divide2/1
  Sum5/1 -> Divide2/2
  Divide2/1 -> Saturation/1
  T_in/1 -> Product/1, Switch/3, MinMax/1
  Saturation/1 -> Product/2
  Multiport Switch/1 -> Product1/1
  Activate?/1 -> Product1/2, Switch/2
  Product1/1 -> Sum6/2, motohawk_probe1/1
  motohawk_fault_action/1 -> Logical Operator/1
  Logical Operator/1 -> Product1/3
  Switch/1 -> Sum6/1
  Product/1 -> Switch/1
  Sum6/1 -> MinMax/2
  MinMax/1 -> T_Out/1

== system cx06_MA/Strategy/Hybrid Control Code/HEV/SOC_RampOut ==
  Torque_In : Inport  OutDataType=sfix(16)  OutScaling=2^0
  SOC : Inport  Port=2  OutDataType=sfix(16)  OutScaling=2^0
  Constant : Constant  OutDataType=sfix(16)  OutScaling=2^0
  Divide : Product  Inputs=*/  OutDataType=sfix(16)  OutScaling=2^-10
  Product : Product  OutDataType=sfix(16)  OutScaling=2^0  RndMeth=Zero
  Relational Operator : RelationalOperator  Operator=>  LogicOutDataTypeMode=boolean  OutDataTypeStr=boolean
  Saturation : Saturate  UpperLimit=1  LowerLimit=0
  Sum : Sum  Inputs=+-+  OutDataType=sfix(16)  OutScaling=2^0
  Switch : Switch  Criteria=u2 ~= 0
  motohawk_calibration : MotoHawk_lib/Calibration & Probing Blocks/motohawk_calibration  nam='AssistSOCRampWidth'  val=5  storage=Calibration  show_more=on  name_source=Use Parameter  data_type=Inherit from 'Default Value'  read_level=1  write_level=1  ovr_cals=on  view_as=Number  enum_struct={'Disabled', 'Enabled'}  vector_style=Wide Row  use_help_units=on  help='Assist ramps out this fast below min'  units='%'  use_header_enum=off  row_header_enum={}  col_header_enum={}  use_min_max=on  min_val=0  max_val=100  use_precision=off  precision=''  gain=1  offset=0  exp=1  use_mototune_group=off  mototune_group=motohawk_vardec_path(gcb)
  motohawk_calibration1 : MotoHawk_lib/Calibration & Probing Blocks/motohawk_calibration  nam='AssistMinSOC'  val=30  storage=Calibration  show_more=on  name_source=Use Parameter  data_type=Inherit from 'Default Value'  read_level=1  write_level=1  ovr_cals=on  view_as=Number  enum_struct={'Disabled', 'Enabled'}  vector_style=Wide Row  use_help_units=on  help='Minimum SOC to assist'  units='%'  use_header_enum=off  row_header_enum={}  col_header_enum={}  use_min_max=on  min_val=0  max_val=100  use_precision=off  precision=''  gain=1  offset=0  exp=1  use_mototune_group=off  mototune_group=motohawk_vardec_path(gcb)
  Torque_Out : Outport  OutDataType=sfix(16)  OutScaling=2^0
  wires:
  SOC/1 -> Sum/1, Relational Operator/1
  motohawk_calibration1/1 -> Sum/2, Relational Operator/2
  motohawk_calibration/1 -> Divide/2, Sum/3
  Sum/1 -> Divide/1
  Relational Operator/1 -> Switch/2
  Divide/1 -> Switch/3
  Constant/1 -> Switch/1
  Torque_In/1 -> Product/1
  Switch/1 -> Saturation/1
  Product/1 -> Torque_Out/1
  Saturation/1 -> Product/2
